simulink model "ldr_dlx01"  (R2022a)
settings: Solver=VariableStepAuto  StartTime=0.0  StopTime=70  RelTol=1e-3
undefined symbols (not defined in the file): cx, cy, r_k, r_yaw
libraries: Solver_SF x2, simulink x2
settings Model: Creator=wenju  LastModifiedBy=wenju

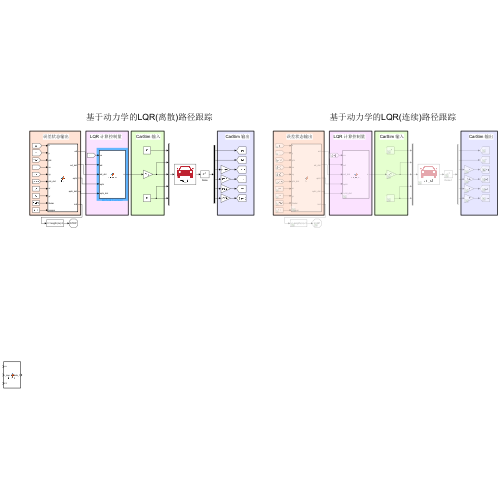
[thumbnail: Simulink's stored preview of the top-level diagram]
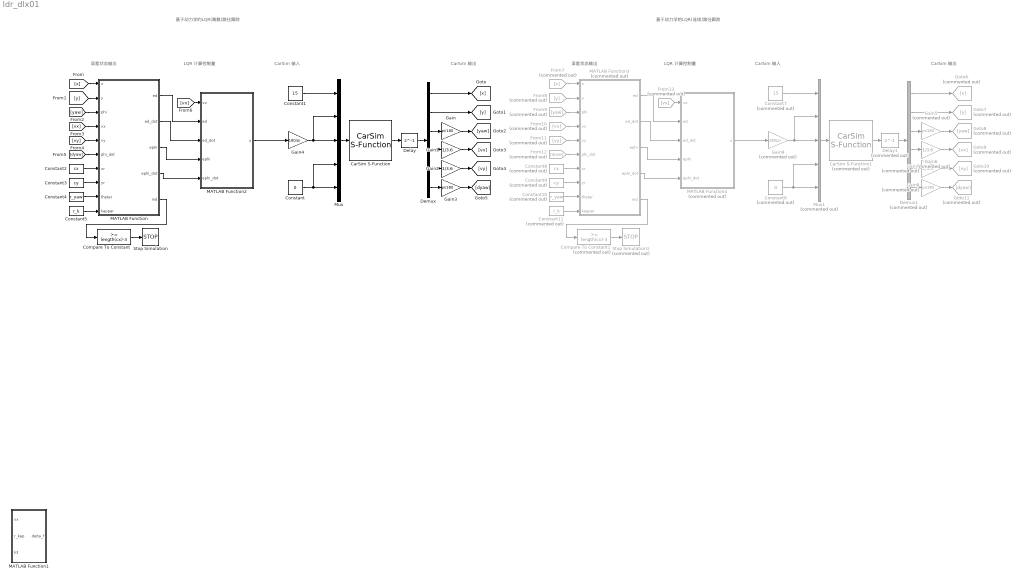
== system ldr_dlx01 ==
  note: 基于动力学的LQR(离散)路径跟踪
  note: CarSim 输出
  note: CarSim 输入
  note: LQR 计算控制量
  note: 误差状态输出
  note: 误差状态输出
  note: CarSim 输出
  note: CarSim 输入
  note: 基于动力学的LQR(连续)路径跟踪
  note: LQR 计算控制量
  CarSim S-Function : Solver_SF/CarSim S-Function  Priority=1  SIMFILE=simfile.sim  Run_RTs=off  vs_state_ind=Run  StopMode_ind=Vehicle Model
  CarSim S-Function1 : Solver_SF/CarSim S-Function  Priority=1  Commented=on  SIMFILE=simfile.sim  Run_RTs=off  vs_state_ind=Run  StopMode_ind=Vehicle Model
  Compare To Constant : simulink/Logic and Bit Operations/Compare To Constant  relop=>=  const=length(cx)-3  OutDataTypeStr=boolean
  Compare To Constant1 : simulink/Logic and Bit Operations/Compare To Constant  Commented=on  relop=>=  const=length(cx)-3  OutDataTypeStr=boolean
  Constant : Constant  Value=0
  Constant1 : Constant  Value=15
  Constant10 : Constant  Commented=on  Value=r_yaw
  Constant11 : Constant  Commented=on  Value=r_k
  Constant2 : Constant  Value=cx
  Constant3 : Constant  Value=cy
  Constant4 : Constant  Value=r_yaw
  Constant5 : Constant  Value=r_k
  Constant6 : Constant  Commented=on  Value=0
  Constant7 : Constant  Commented=on  Value=15
  Constant8 : Constant  Commented=on  Value=cx
  Constant9 : Constant  Commented=on  Value=cy
  Delay : Delay  DelayLength=1  InitialCondition=0  UseCircularBuffer=on
  Delay1 : Delay  Commented=on  DelayLength=1  InitialCondition=0  UseCircularBuffer=on
  Demux : Demux  Outputs=6
  Demux1 : Demux  Commented=on  Outputs=6
  From10 : From  Commented=on  GotoTag=vx
  From11 : From  Commented=on  GotoTag=vy
  From12 : From  Commented=on  GotoTag=dyaw
  From13 : From  Commented=on  GotoTag=vx
  From7 : From  Commented=on  GotoTag=x
  From8 : From  Commented=on  GotoTag=y
  From9 : From  Commented=on  GotoTag=yaw
  Gain : Gain  Gain=pi/180
  Gain1 : Gain  Gain=1/3.6
  Gain2 : Gain  Gain=1/3.6
  Gain3 : Gain  Gain=pi/180
  Gain4 : Gain  Gain=180/pi
  Gain5 : Gain  Commented=on  Gain=pi/180
  Gain6 : Gain  Commented=on  Gain=1/3.6
  Gain7 : Gain  Commented=on  Gain=1/3.6
  Gain8 : Gain  Commented=on  Gain=pi/180
  Gain9 : Gain  Commented=on  Gain=180/pi
  Goto10 : Goto  Commented=on  GotoTag=vy
  Goto11 : Goto  Commented=on  GotoTag=dyaw
  Goto6 : Goto  Commented=on  GotoTag=x
  Goto7 : Goto  Commented=on  GotoTag=y
  Goto8 : Goto  Commented=on  GotoTag=yaw
  Goto9 : Goto  Commented=on  GotoTag=vx
  MATLAB Function : MATLAB Function  TreatAsAtomicUnit=on
  MATLAB Function1 : MATLAB Function  TreatAsAtomicUnit=on
  MATLAB Function2 : MATLAB Function  TreatAsAtomicUnit=on
  MATLAB Function3 : MATLAB Function  Commented=on  TreatAsAtomicUnit=on
  MATLAB Function4 : MATLAB Function  Commented=on  TreatAsAtomicUnit=on
  Mux : Mux  Inputs=5
  Mux1 : Mux  Commented=on  Inputs=5
  Stop Simulation : Stop
  Stop Simulation1 : Stop  Commented=on
  wires:
  CarSim S-Function/1 -> Delay/1
  Delay/1 -> Demux/1
  Mux/1 -> CarSim S-Function/1
  Demux/1 -> [x]
  Demux/2 -> [y]
  Demux/3 -> Gain/1
  Gain/1 -> [yaw]
  Demux/4 -> Gain1/1
  Gain1/1 -> [vx]
  Demux/5 -> Gain2/1
  Gain2/1 -> [vy]
  Demux/6 -> Gain3/1
  Gain3/1 -> [dyaw]
  Constant/1 -> Mux/4, Mux/5
  Gain4/1 -> Mux/2, Mux/3
  Constant1/1 -> Mux/1
  [x] -> MATLAB Function/1(x)
  [y] -> MATLAB Function/2(y)
  [yaw] -> MATLAB Function/3(phi)
  [vx] -> MATLAB Function/4(vx)
  [vy] -> MATLAB Function/5(vy)
  [dyaw] -> MATLAB Function/6(phi_dot)
  Constant2/1 -> MATLAB Function/7(xr)
  Constant3/1 -> MATLAB Function/8(yr)
  Constant4/1 -> MATLAB Function/9(thetar)
  Constant5/1 -> MATLAB Function/10(kappar)
  MATLAB Function/5(ind) -> Compare To Constant/1
  Compare To Constant/1 -> Stop Simulation/1
  [vx] -> MATLAB Function2/1(vx)
  MATLAB Function/1(ed) -> MATLAB Function2/2(ed)
  MATLAB Function/2(ed_dot) -> MATLAB Function2/3(ed_dot)
  MATLAB Function/3(ephi) -> MATLAB Function2/4(ephi)
  MATLAB Function/4(ephi_dot) -> MATLAB Function2/5(ephi_dot)
  MATLAB Function2/1(u) -> Gain4/1
  Gain9/1 -> Mux1/2, Mux1/3
  Mux1/1 -> CarSim S-Function1/1
  CarSim S-Function1/1 -> Delay1/1
  From9/1 -> MATLAB Function3/3(phi)
  MATLAB Function3/3(ephi) -> MATLAB Function4/4(ephi)
  From10/1 -> MATLAB Function3/4(vx)
  MATLAB Function3/2(ed_dot) -> MATLAB Function4/3(ed_dot)
  Constant11/1 -> MATLAB Function3/10(kappar)
  MATLAB Function3/1(ed) -> MATLAB Function4/2(ed)
  From7/1 -> MATLAB Function3/1(x)
  Gain8/1 -> Goto11/1
  Demux1/2 -> Goto7/1
  Constant8/1 -> MATLAB Function3/7(xr)
  Compare To Constant1/1 -> Stop Simulation1/1
  Constant7/1 -> Mux1/1
  Demux1/5 -> Gain7/1
  Gain7/1 -> Goto10/1
  Demux1/6 -> Gain8/1
  MATLAB Function3/5(ind) -> Compare To Constant1/1
  MATLAB Function4/1(u) -> Gain9/1
  Constant10/1 -> MATLAB Function3/9(thetar)
  Constant6/1 -> Mux1/4, Mux1/5
  Demux1/1 -> Goto6/1
  From13/1 -> MATLAB Function4/1(vx)
  From8/1 -> MATLAB Function3/2(y)
  From12/1 -> MATLAB Function3/6(phi_dot)
  Demux1/3 -> Gain5/1
  From11/1 -> MATLAB Function3/5(vy)
  Gain6/1 -> Goto9/1
  MATLAB Function3/4(ephi_dot) -> MATLAB Function4/5(ephi_dot)
  Constant9/1 -> MATLAB Function3/8(yr)
  Demux1/4 -> Gain6/1
  Gain5/1 -> Goto8/1
  Delay1/1 -> Demux1/1

== matlab function ldr_dlx01/MATLAB Function1 ==
  data: vx input; deita_f output; r_kap input; k3 input
function deita_f  = findPoint(vx,r_kap,k3)



% e_X=[ed;ed_dot;ephi; ephi_dot];


% 车辆参数
cf = -148970;
cr = -82204;
m = 1412;
% Iz=1536.7;
lf=1.015;
lr=2.910-1.015;


v=vx+0.05;


deita_f=r_kap*(lf+lr-lr*k3-(m*v*v/(lf+lr))*(lr/cf+(lf/cr)*k3-lf/cr));

end

== matlab function ldr_dlx01/MATLAB Function ==
  data: x input; ed output; y input; phi input; vx input; vy input; phi_dot input; xr input; yr input; thetar input; kappar input; ed_dot output; ephi output; ephi_dot output; ind output
function [ed,ed_dot,ephi,ephi_dot,ind] = fcn(x,y,phi, vx,vy,phi_dot,xr,yr,thetar,kappar)
    %寻找匹配点
    n=length(xr);
    d_min=(x-xr(1))^2+(y-yr(1))^2;
    min=1;
    for i=1:n
        d=(x-xr(i))^2+(y-yr(i))^2;
        if d<d_min
            d_min=d;
            min=i;
        end
    end
    ind=min;

    %计算状态方程中的状态向量
    tor=[cos(thetar(ind));sin(thetar(ind))];
    nor=[-sin(thetar(ind));cos(thetar(ind))];

    d_err=[x-xr(ind);y-yr(ind)]; 

    ed=nor'*d_err;                  %求取状态向量中的第一个 ed
    
    projection_point_thetar=thetar(ind); %百度apollo

    ed_dot=vy*cos(phi-projection_point_thetar)+vx*sin(phi-projection_point_thetar);%求取状态向量中的第二个 ed的导数

    ephi=sin(phi-projection_point_thetar);    %求取状态向量中的第三个 efai

    s_dot=vx*cos(phi-projection_point_thetar)-vy*sin(phi-projection_point_thetar);
    s_dot=s_dot/(1-kappar(ind)*ed);
    
    ephi_dot=phi_dot-kappar(ind)*s_dot;%求取状态向量中的第四个 efai 的倒数


end

== matlab function ldr_dlx01/MATLAB Function2 ==
  data: vx input; ed input; u output; ed_dot input; ephi input; ephi_dot input
% 首先在参考轨迹上搜索离当前车辆位置最近的点
function u   = findPoint(vx,ed,ed_dot,ephi, ephi_dot)
e_X=[ed;ed_dot;ephi; ephi_dot];

% 车辆参数
    cf = -79127;
    cr = -79127;
    m = 1235.9;
    Iz=1343.1;
    lf=1.3;
    lr=2.6-1.3;
% 离散化采样时
    T=0.05; 

v=vx+0.05;    % 分母不能为0，故加上很小数
% 离散化之前的状态空间方程的矩阵系数 A,B
 a1=[0,          1,                  0,                  0;
     0,    (cf+cr)/(m*v),       -(cf+cr)/m,     (lf*cf-lr*cr)/(m*v);
     0,          0,                 0,                   1;
     0,(lf*cf-lr*cr)/(Iz*v),-(lf*cf-lr*cr)/Iz,(lf^2*cf+lr^2*cr)/(Iz*v)];

 b1=[   0;
      -cf/m;
        0;
    -lf*cf/Iz];
% 离散化之后的状态空间方程的矩阵系数 A,B
 A = (eye(4)-a1*T/2)\(eye(4)+a1*T/2);  %中点欧拉法离散化
 B = T*b1;                             %向前欧拉法离散化

% 由状态方程矩阵系数，计算K
    Q=1 *[30,0,0,0;
        0,5,0,0;
        0,0,5,0
        0,0,0,1];
    R=2;

% 终止条件定义
iter_max = 500;         %最大迭代次数
epsilon = 0.01;         %容忍的最大误差

% 求解反馈增益 K
P_old = Q;
for i = 1:iter_max
    P_new = A' * P_old * A - (A' * P_old * B) / (R + B' * P_old * B) *( B' * P_old * A) +Q;
    if abs(P_new - P_old) <= epsilon
        break
    else
        P_old = P_new; 
    end
end

P = P_new;
K = (B' * P * B + R) \ (B' * P * A);  % 2行3列

% 获得速度误差量、前轮转角误差量两个控制量
u = -K * e_X;  % 2行1列

end

== matlab function ldr_dlx01/MATLAB Function3 ==
  data: x input; ed output; y input; phi input; vx input; vy input; phi_dot input; xr input; yr input; thetar input; kappar input; ed_dot output; ephi output; ephi_dot output; ind output
function [ed,ed_dot,ephi,ephi_dot,ind] = fcn(x,y,phi, vx,vy,phi_dot,xr,yr,thetar,kappar)
    %寻找匹配点
    n=length(xr);
    d_min=(x-xr(1))^2+(y-yr(1))^2;
    min=1;
    for i=1:n
        d=(x-xr(i))^2+(y-yr(i))^2;
        if d<d_min
            d_min=d;
            min=i;
        end
    end
    ind=min;

    %计算状态方程中的状态向量
    tor=[cos(thetar(ind));sin(thetar(ind))];
    nor=[-sin(thetar(ind));cos(thetar(ind))];

    d_err=[x-xr(ind);y-yr(ind)]; 

    ed=nor'*d_err;                  %求取状态向量中的第一个 ed
    
    projection_point_thetar=thetar(ind); %百度apollo

    ed_dot=vy*cos(phi-projection_point_thetar)+vx*sin(phi-projection_point_thetar);%求取状态向量中的第二个 ed的导数

    ephi=sin(phi-projection_point_thetar);    %求取状态向量中的第三个 efai

    s_dot=vx*cos(phi-projection_point_thetar)-vy*sin(phi-projection_point_thetar);
    s_dot=s_dot/(1-kappar(ind)*ed);
    
    ephi_dot=phi_dot-kappar(ind)*s_dot;%求取状态向量中的第四个 efai 的倒数


end

== matlab function ldr_dlx01/MATLAB Function4 ==
  data: vx input; ed input; u output; ed_dot input; ephi input; ephi_dot input
function u   = findPoint(vx,ed,ed_dot,ephi, ephi_dot)
% 状态量    
    e_X=[ed;ed_dot;ephi; ephi_dot];

% 车辆参数
    cf = -79127;
    cr = -79127;
    m = 1235.9;
    Iz = 1343.1;
    lf = 1.3;
    lr = 2.6-1.3;

    v=vx+0.05;   %防止分母为0
% 离散化之前的状态空间方程的矩阵系数 A,B
    a1=[0,          1,                  0,                  0;
        0,    (cf+cr)/(m*v),       -(cf+cr)/m,     (lf*cf-lr*cr)/(m*v);
        0,          0,                 0,                   1;
        0,(lf*cf-lr*cr)/(Iz*v),-(lf*cf-lr*cr)/Iz,(lf^2*cf+lr^2*cr)/(Iz*v)];
    
    b1=[   0;
         -cf/m;
           0;
       -lf*cf/Iz];

% 权重矩阵 Q,R
    Q=1 *[30,0,0,0;
          0,5,0,0;
          0,0,10,0
          0,0,0,1];
    R=2;

coder.extrinsic('lqr');
K=[0 0 0 0];
K=lqr(a1,b1,Q,R);

% 获得速度误差量、前轮转角误差量两个控制量
u = -K * e_X;  % 2行1列
 
end










% cf = -148970;
% cr = -82204;
% m = 1412;
% Iz=1536.7;
% lf=1.015;
% lr=2.910-1.015;

% 根据百度Apolo，计算横向误差
% latError = y_error*cos(heading_r) - x_error*sin(heading_r);

% k3=K(3);
